simulink model "FDIBenchMark"  (Simulink 8.4)
settings: Solver=ode45  StartTime=0.0  StopTime=4400  FixedStep=Ts  RelTol=1e-12
InitFcn:
  | FDIBenchMarkData
values from neighbouring files (symbols this model uses):
  a = 2.2    [FDIBenchMarkData.m]
  Addt = [-(B_dt+B_r)/J_r B_dt/N_g/J_r -K_dt/J_r; eta_dt*B_dt/N_g/J_g -(eta_dt*B_dt/N_g^2+B_g)/J_g eta_dt*K_dt/N_g/J_g; 1 -1/N_g 0]    [FDIBenchMarkData.m]
  Addt2 = [-(B_dt+B_r)/J_r B_dt/N_g/J_r -K_dt/J_r; eta_dt2*B_dt/N_g/J_g -(eta_dt2*B_dt/N_g^2+B_g)/J_g eta_dt2*K_dt/N_g/J_g; 1 -1/N_g 0]    [FDIBenchMarkData.m]
  alpha = 0.1    [FDIBenchMarkData.m]
  alpha_gc = 50    [FDIBenchMarkData.m]
  Bddt = [1/J_r 0; 0 -1/J_g;0 0]    [FDIBenchMarkData.m]
  Bddt2 = [1/J_r 0; 0 -1/J_g;0 0]    [FDIBenchMarkData.m]
  Cddt = [1 0 0;0 1 0]    [FDIBenchMarkData.m]
  Constant_Beta_1_m1 = 5    [FDIBenchMarkData.m]
  Constant_Beta_3_m1 = 10    [FDIBenchMarkData.m]
  Constant_Omega_r_m1 = 1.4    [FDIBenchMarkData.m]
  Constant_tau_gc = 100    [FDIBenchMarkData.m]
  eta_gc = 0.98    [FDIBenchMarkData.m]
  Gain_Beta_2_m2 = 1.2    [FDIBenchMarkData.m]
  Gain_Omega_r_m2 = 1.1    [FDIBenchMarkData.m]
  H = 87    [FDIBenchMarkData.m]
  k = 4.7    [FDIBenchMarkData.m]
  K_i = 1    [FDIBenchMarkData.m]
  K_opt = .5* rho* pi*R^2*eta_dt*R^3*0.4554/(N_g*8)^3    (= 1.21708013189)    [FDIBenchMarkData.m]
  K_p = 4    [FDIBenchMarkData.m]
  L = acker(A', C', vpe)'    [FDIBenchMarkData.m]
  Lungime_Fereastra = 512    [FDIBenchMarkData.m]
  Lungime_Fereastra_2 = 5    [FDIBenchMarkData.m]
  Lungime_Fereastra_3 = 100    [FDIBenchMarkData.m]
  m = 1+alpha*(alpha-1)*R^2/(8*H^2)    (= 0.995085835315)    [FDIBenchMarkData.m]
  m_Beta = 0    [FDIBenchMarkData.m]
  m_omega_g = 0    [FDIBenchMarkData.m]
  m_omega_r = 0    [FDIBenchMarkData.m]
  m_P_g = 0    [FDIBenchMarkData.m]
  m_tau_g = 0    [FDIBenchMarkData.m]
  m_vw = 1.5    [FDIBenchMarkData.m]
  Omega_delta = 15    [FDIBenchMarkData.m]
  omega_n = 11.11    [FDIBenchMarkData.m]
  Omega_nom = 162    [FDIBenchMarkData.m]
  P_r = 4.8e6    (= 4800000)    [FDIBenchMarkData.m]
  R = 57.5    [FDIBenchMarkData.m]
  r = D_rotor/2    (= 57.5)    [FDIBenchMarkData.m]
  r0 = 1.5    [FDIBenchMarkData.m]
  rho = 1.225    [FDIBenchMarkData.m]
  seed = ceil(seed)    [FDIBenchMarkData.m]
  sigma_Beta = 0.2    [FDIBenchMarkData.m]
  sigma_omega_g = 0.05    [FDIBenchMarkData.m]
  sigma_omega_r = 0.004*2*pi    (= 0.0251327412287)    [FDIBenchMarkData.m]
  sigma_P_g = 1e3    (= 1000)    [FDIBenchMarkData.m]
  sigma_tau_g = 90    [FDIBenchMarkData.m]
  sigma_vm = 0.5    [FDIBenchMarkData.m]
  T_sample = 0.05    [FDIBenchMarkData.m]
  Ts = 1/100    (= 0.01)    [FDIBenchMarkData.m]
  turb_int = Turbulence_intensity    (= 12)    [FDIBenchMarkData.m]
  xi = 0.6    [FDIBenchMarkData.m]
undefined symbols (not defined in the file or in its folder): A, Apb, Apb1, Apb2, B, Bpb, Bpb1, Bpb2, C, Cpb, Cpb1, Cpb2, Cq, Fa, Fb, u0
undefined symbols (not defined in the file): turbulence_seeds
(part 1 of 2)
settings Model: Creator=peodg  LastModifiedBy=ALEXANDRU
settings SolverCC: MaxConsecutiveZCs=1e6
settings OptimizationCC: InitFltsAndDblsToZero=on
settings SFSimCC: SimParseCustomCode=off

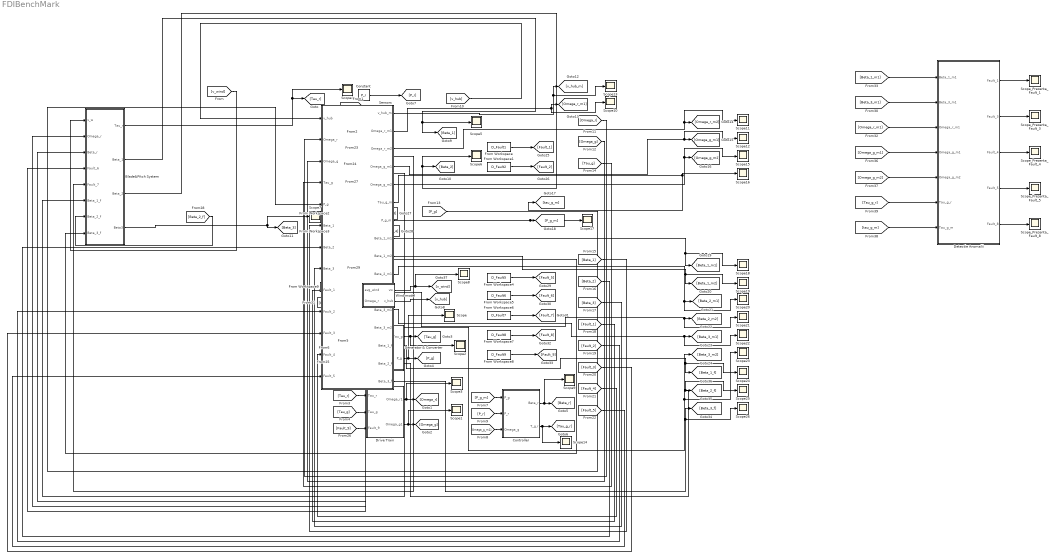
== system FDIBenchMark ==
  Blade&Pitch System : Subsystem
  Constant : Constant  Value=P_r
  Controller : Subsystem
  Detectie Anomalii : Subsystem
  Drive Train : Subsystem
  From Workspace : FromWorkspace  VariableName=D_Fault1  SampleTime=Ts
  From Workspace1 : FromWorkspace  VariableName=D_Fault2  SampleTime=Ts
  From Workspace2 : FromWorkspace  VariableName=D_Fault3  SampleTime=Ts
  From Workspace3 : FromWorkspace  VariableName=D_Fault4  SampleTime=Ts
  From Workspace4 : FromWorkspace  VariableName=D_Fault5  SampleTime=Ts
  From Workspace5 : FromWorkspace  VariableName=D_Fault6  SampleTime=Ts
  From Workspace6 : FromWorkspace  VariableName=D_Fault7  SampleTime=Ts
  From Workspace7 : FromWorkspace  VariableName=D_Fault8  SampleTime=Ts
  From Workspace8 : FromWorkspace  VariableName=D_Fault9  SampleTime=Ts
  From Workspace9 : FromWorkspace  VariableName=D_v_wind
  Generator & Converter : Subsystem
  Scope{,1..26} (27 alike) : Scope
      Scope settings: YMin=200000  YMax=1.2e+06  SaveName=P_g  SampleInput=on  SampleTime=Ts
      Scope1 settings: YMin=64  YMax=66.25  SaveName=Oemga_g1  SampleInput=on  SampleTime=Ts
      Scope10 settings: YMin=1.1  YMax=2.4  SaveName=Omega_r_m1  SampleInput=on  SampleTime=Ts
      Scope11 settings: YMin=-1  YMax=1  SaveName=Omega_r_m2  SampleInput=on  SampleTime=Ts
      Scope12 settings: YMin=-1  YMax=1  SaveName=Omega_g_m1  SampleInput=on  SampleTime=Ts
      Scope13 settings: YMin=-1  YMax=1  SaveName=v_hub_m  SampleInput=on  SampleTime=Ts
      Scope14 settings: YMin=-2.5  YMax=20  SaveName=T_g_r  SampleInput=on  SampleTime=Ts
      Scope15 settings: YMin=-1  YMax=1  SaveName=Omega_g_m2  SampleInput=on  SampleTime=Ts
      Scope16 settings: YMin=-1  YMax=1  SaveName=Tau_g_m  SampleInput=on  SampleTime=Ts
      Scope17 settings: YMin=-1  YMax=1  SaveName=P_g_m  SampleInput=on  SampleTime=Ts
      Scope18 settings: YMin=-1  YMax=1  SaveName=Beta_1_m1  SampleInput=on  SampleTime=Ts
      Scope19 settings: YMin=-1  YMax=1  SaveName=Beta_1_m2  SampleInput=on  SampleTime=Ts
      Scope2 settings: YMin=29400  YMax=29875  SaveName=Tau_g  SampleInput=on  SampleTime=Ts
      Scope20 settings: YMin=-1  YMax=1  SaveName=Beta_2_m1  SampleInput=on  SampleTime=Ts
      Scope21 settings: YMin=-1  YMax=1  SaveName=Beta_2_m2  SampleInput=on  SampleTime=Ts
      Scope22 settings: YMin=-1  YMax=1  SaveName=Beta_3_m1  SampleInput=on  SampleTime=Ts
      Scope23 settings: YMin=-1  YMax=1  SaveName=Beta_3_m2  SampleInput=on  SampleTime=Ts
      Scope24 settings: YMin=-1  YMax=1  SaveName=Beta_1_f  SampleInput=on  SampleTime=Ts
      Scope25 settings: YMin=-1  YMax=1  SaveName=Beta_2_f  SampleInput=on  SampleTime=Ts
      Scope26 settings: YMin=-1  YMax=1  SaveName=Beta_3_f  SampleInput=on  SampleTime=Ts
      Scope3 settings: YMin=0.62  YMax=0.69  SaveName=Omega_r1  SampleInput=on  SampleTime=Ts
      Scope4 settings: YMin=-1e+006  YMax=6e+006  SaveName=Tau_r  SampleInput=on  SampleTime=Ts
      Scope5 settings: YMin=-3  YMax=8  SaveName=Beta1  SampleInput=on  SampleTime=Ts
      Scope6 settings: YMin=-0.3  YMax=0.3  SaveName=Beta  SampleInput=on  SampleTime=Ts
      Scope7 settings: YMin=-0.25  YMax=0.35  SaveName=Beta3  SampleInput=on  SampleTime=Ts
      Scope8 settings: YMin=3  YMax=18  SaveName=Vw  SampleInput=on  SampleTime=Ts
      Scope9 settings: YMin=-1  YMax=1  SaveName=Beta_r  SampleInput=on  SampleTime=Ts
  Scope_Prezenta_Fault_{1,3..5,8} (5 alike) : Scope
      Scope_Prezenta_Fault_1 settings: YMin=-0  YMax=2  SaveName=ScopeData5
      Scope_Prezenta_Fault_3 settings: YMin=-0.03  YMax=0.02
      Scope_Prezenta_Fault_4 settings: YMin=-0.03  YMax=0.02
      Scope_Prezenta_Fault_5 settings: YMin=-0.03  YMax=0.02  SaveName=ScopeData8
      Scope_Prezenta_Fault_8 settings: YMin=-0.03  YMax=0.02  SaveName=ScopeData9
  Sensors : Subsystem
  Wind model : Subsystem
  wires:
  [v_wind] -> Blade&Pitch System/1(v_w)
  [Omega_r] -> Blade&Pitch System/2(Omega_r)
  [Beta_r] -> Blade&Pitch System/3(Beta_r)
  [Tau_r] -> Drive Train/1(Tau_r)
  [Tau_g] -> Drive Train/2(Tau_g)
  Drive Train/1(Omega_r1) -> [Omega_r], Scope3/1
  [Tau_g_r] -> Generator & Converter/1(Tau_g,r)
  [Omega_g] -> Generator & Converter/2(Omega_g)
  Generator & Converter/1(Tau_g) -> [Tau_g], Scope2/1
  Generator & Converter/2(P_g) -> [P_g], Scope/1
  [P_g_m] -> Controller/1(P_g)
  [Omega_g_m1] -> Controller/3(Omega_g)
  Controller/1(Beta_r) -> [Beta_r], Scope9/1
  Controller/2(T_g,r) -> [Tau_g_r], Scope14/1
  [P_r] -> Controller/2(P_r)
  Constant/1 -> [P_r]
  Sensors/1(v_hub_m) -> [v_hub_m], Scope13/1
  Sensors/2(Omega_r_m1) -> [Omega_r_m1], Scope10/1
  Sensors/3(Omega_r_m2) -> [Omega_r_m2], Scope11/1
  Sensors/4(Omega_g_m1) -> [Omega_g_m1], Scope12/1
  Sensors/5(Omega_g_m2) -> Scope15/1, [Omega_g_m2]
  Sensors/6(Tau_g_m) -> [tau_g_m], Scope16/1
  Sensors/7(P_g_m) -> [P_g_m], Scope17/1
  Sensors/8(Beta_1_m1) -> [Beta_1_m1], Scope18/1
  Sensors/9(Beta_1_m2) -> [Beta_1_m2], Scope19/1
  Sensors/10(Beta_2_m1) -> [Beta_2_m1], Scope20/1
  Sensors/11(Beta_2_m2) -> [Beta_2_m2], Scope21/1
  Sensors/12(Beta_3_m1) -> [Beta_3_m1], Scope22/1
  Sensors/13(Beta_3_m2) -> [Beta_3_m2], Scope23/1
  [v_hub] -> Sensors/1(v_hub)
  [Omega_r] -> Sensors/2(Omega_r)
  [Omega_g] -> Sensors/3(Omega_g)
  [Tau_g] -> Sensors/4(Tau_g)
  [P_g] -> Sensors/5(P_g)
  [Beta_1] -> Sensors/6(Beta_1)
  [Beta_2] -> Sensors/7(Beta_2)
  [Beta_3] -> Sensors/8(Beta_3)
  [Fault_1] -> Sensors/9(Fault_1)
  [Fault_2] -> Sensors/10(Fault_2)
  [Fault_3] -> Sensors/11(Fault_3)
  [Fault_4] -> Sensors/12(Fault_4)
  [Fault_5] -> Sensors/13(Fault_5)
  [Fault_6] -> Blade&Pitch System/4(Fault_6)
  [Fault_7] -> Blade&Pitch System/5(Fault_7)
  [Fault_8] -> Generator & Converter/3(Fault_8)
  [Fault_9] -> Drive Train/3(Fault_9)
  From Workspace8/1 -> [Fault_9]
  From Workspace7/1 -> [Fault_8]
  From Workspace6/1 -> [Fault_7]
  From Workspace5/1 -> [Fault_6]
  From Workspace4/1 -> [Fault_5]
  From Workspace3/1 -> [Fault_4]
  From Workspace2/1 -> [Fault_3]
  From Workspace1/1 -> [Fault_2]
  From Workspace/1 -> [Fault_1]
  Drive Train/2(Omega_g1) -> [Omega_g], Scope1/1
  Sensors/16(Beta_3_f) -> [Beta_3_f], Scope26/1
  Sensors/15(Beta_2_f) -> [Beta_2_f], Scope25/1
  Sensors/14(Beta_1_f) -> [Beta_1_f], Scope24/1
  [Beta_1_f] -> Blade&Pitch System/6(Beta_1_f)
  [Beta_2_f] -> Blade&Pitch System/7(Beta_2_f)
  [Beta_3_f] -> Blade&Pitch System/8(Beta_3_f)
  Blade&Pitch System/4(Beta3) -> [Beta_3], Scope7/1
  Blade&Pitch System/3(Beta_2) -> [Beta_2], Scope6/1
  Blade&Pitch System/2(Beta_1) -> [Beta_1], Scope5/1
  Blade&Pitch System/1(Tau_r) -> [Tau_r], Scope4/1
  Wind model/1(vw) -> [v_wind], Scope8/1
  Wind model/2(v_hub) -> [v_hub]
  [Omega_r] -> Wind model/2(Omega_r)
  From Workspace9/1 -> Wind model/1(avg_wind)
  [Beta_1_m1] -> Detectie Anomalii/1(Beta_1_m1)
  [Beta_3_m1] -> Detectie Anomalii/2(Beta_3_m1)
  [Omega_r_m1] -> Detectie Anomalii/3(Omega_r_m1)
  [Omega_g_m1] -> Detectie Anomalii/4(Omega_g_m1)
  [Omega_g_m2] -> Detectie Anomalii/5(Omega_g_m2)
  [Tau_g_r] -> Detectie Anomalii/6(Tau_g_r)
  [tau_g_m] -> Detectie Anomalii/7(Tau_g_m)
  Detectie Anomalii/1(Fault_1) -> Scope_Prezenta_Fault_1/1
  Detectie Anomalii/2(Fault_3) -> Scope_Prezenta_Fault_3/1
  Detectie Anomalii/3(Fault_4) -> Scope_Prezenta_Fault_4/1
  Detectie Anomalii/4(Fault_5) -> Scope_Prezenta_Fault_5/1
  Detectie Anomalii/5(Fault_8) -> Scope_Prezenta_Fault_8/1

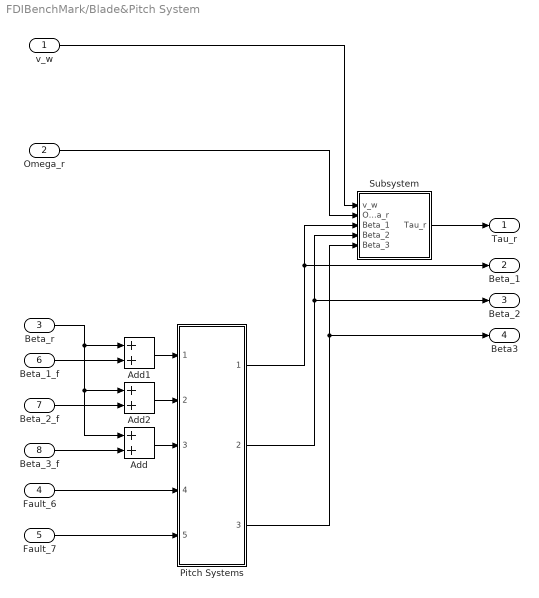
== system FDIBenchMark/Blade&Pitch System ==
  v_w : Inport
  Omega_r : Inport  Port=2
  Beta_r : Inport  Port=3
  Fault_6 : Inport  Port=4
  Fault_7 : Inport  Port=5
  Beta_1_f : Inport  Port=6
  Beta_2_f : Inport  Port=7
  Beta_3_f : Inport  Port=8
  Add : Sum
  Add1 : Sum
  Add2 : Sum
  Pitch Systems : Subsystem
  Subsystem : Subsystem
  Tau_r : Outport
  Beta_1 : Outport  Port=2
  Beta_2 : Outport  Port=3
  Beta3 : Outport  Port=4
  wires:
  Pitch Systems/1(Beta_1) -> Subsystem/3(Beta_1), Beta_1/1
  Pitch Systems/2(Beta_2) -> Subsystem/4(Beta_2), Beta_2/1
  Pitch Systems/3(Beta_3) -> Subsystem/5(Beta_3), Beta3/1
  Subsystem/1(Tau_r) -> Tau_r/1
  v_w/1 -> Subsystem/1(v_w)
  Omega_r/1 -> Subsystem/2(Omega_r)
  Fault_6/1 -> Pitch Systems/4(Fault_6)
  Fault_7/1 -> Pitch Systems/5(Fault_7)
  Add/1 -> Pitch Systems/3(Beta_r3)
  Add1/1 -> Pitch Systems/1(Beta_r1)
  Add2/1 -> Pitch Systems/2(Beta_r2)
  Beta_3_f/1 -> Add/2
  Beta_2_f/1 -> Add2/2
  Beta_1_f/1 -> Add1/2
  Beta_r/1 -> Add1/1, Add2/1, Add/1

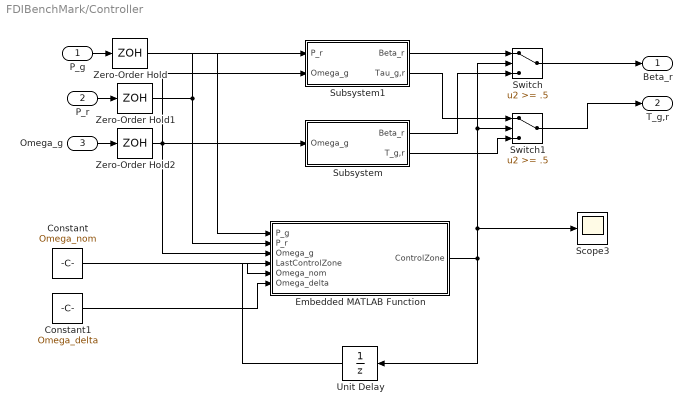
== system FDIBenchMark/Controller ==
  P_g : Inport
  P_r : Inport  Port=2
  Omega_g : Inport  Port=3
  Constant : Constant  Value=Omega_nom
  Constant1 : Constant  Value=Omega_delta
  Embedded MATLAB Function : MATLAB Function  TreatAsAtomicUnit=on
  Scope3 : Scope
      settings: YMin=0.62  YMax=0.69  SaveName=Omega_r  SampleInput=on  SampleTime=Ts
  Subsystem : Subsystem
  Subsystem1 : Subsystem
  Switch : Switch  Threshold=.5
  Switch1 : Switch  Threshold=.5
  Unit Delay : UnitDelay  SampleTime=Ts
  Zero-Order Hold : ZeroOrderHold  SampleTime=Ts
  Zero-Order Hold1 : ZeroOrderHold  SampleTime=Ts
  Zero-Order Hold2 : ZeroOrderHold  SampleTime=Ts
  Beta_r : Outport
  T_g,r : Outport  Port=2
  wires:
  Embedded MATLAB Function/1(ControlZone) -> Unit Delay/1, Switch/2, Switch1/2, Scope3/1
  Unit Delay/1 -> Embedded MATLAB Function/4(LastControlZone)
  P_g/1 -> Zero-Order Hold/1
  P_r/1 -> Zero-Order Hold1/1
  Omega_g/1 -> Zero-Order Hold2/1
  Switch/1 -> Beta_r/1
  Switch1/1 -> T_g,r/1
  Subsystem1/1(Beta_r) -> Switch/1
  Subsystem/1(Beta_r) -> Switch/3
  Subsystem1/2(Tau_g,r) -> Switch1/1
  Subsystem/2(T_g,r) -> Switch1/3
  Constant/1 -> Embedded MATLAB Function/5(Omega_nom)
  Constant1/1 -> Embedded MATLAB Function/6(Omega_delta)
  Zero-Order Hold/1 -> Embedded MATLAB Function/1(P_g)
  Zero-Order Hold1/1 -> Subsystem1/1(P_r), Embedded MATLAB Function/2(P_r)
  Zero-Order Hold2/1 -> Embedded MATLAB Function/3(Omega_g), Subsystem1/2(Omega_g), Subsystem/1(Omega_g)

== system FDIBenchMark/Detectie Anomalii ==
  Beta_1_m1 : Inport
  Beta_3_m1 : Inport  Port=2
  Omega_r_m1 : Inport  Port=3
  Omega_g_m1 : Inport  Port=4
  Omega_g_m2 : Inport  Port=5
  Tau_g_r : Inport  Port=6
  Tau_g_m : Inport  Port=7
  Detectie Fault_1 : Subsystem
  Detectie Fault_3 : Subsystem
  Detectie Fault_4 : Subsystem
  Detectie Fault_5 : Subsystem
  Detectie Fault_8 : Subsystem
  Fault_1 : Outport
  Fault_3 : Outport  Port=2
  Fault_4 : Outport  Port=3
  Fault_5 : Outport  Port=4
  Fault_8 : Outport  Port=5
  wires:
  Tau_g_m/1 -> Detectie Fault_8/2(Tau_g_m)
  Omega_g_m2/1 -> Detectie Fault_5/2(Omega_g_m2)
  Detectie Fault_5/1(Prezenta_Fault_5) -> Fault_5/1
  Omega_g_m1/1 -> Detectie Fault_5/1(Omega_g_m1)
  Beta_1_m1/1 -> Detectie Fault_1/1(Beta_1_m1)
  Detectie Fault_3/1(Prezenta_Fault_3) -> Fault_3/1
  Detectie Fault_4/1(Prezenta_Fault_4) -> Fault_4/1
  Omega_r_m1/1 -> Detectie Fault_4/1(Omega_r_m1)
  Detectie Fault_1/1(Prezenta_Fault_1) -> Fault_1/1
  Beta_3_m1/1 -> Detectie Fault_3/1(Beta_3_m1)
  Detectie Fault_8/1(Prezenta_Fault_8) -> Fault_8/1
  Tau_g_r/1 -> Detectie Fault_8/1(Tau_g_r)

== system FDIBenchMark/Drive Train ==
  Tau_r : Inport
  Tau_g : Inport  Port=2
  Fault_9 : Inport  Port=3
  Add : Sum
  Demux1 : Demux  Outputs=2
  Gain : Gain  Gain=Addt  Multiplication=Matrix(K*u)
  Gain1 : Gain  Gain=Bddt  Multiplication=Matrix(K*u)
  Gain2 : Gain  Gain=Cddt  Multiplication=Matrix(K*u)
  Gain3 : Gain  Gain=Addt2  Multiplication=Matrix(K*u)
  Gain4 : Gain  Gain=Bddt2  Multiplication=Matrix(K*u)
  Integrator : Integrator  InitialCondition=[1 100 0]
  Mux : Mux  Inputs=2
  Switch1 : Switch  Threshold=0.5
  Switch2 : Switch  Threshold=0.5
  Omega_r1 : Outport
  Omega_g1 : Outport  Port=2
  wires:
  Tau_r/1 -> Mux/1
  Tau_g/1 -> Mux/2
  Integrator/1 -> Gain2/1, Gain/1, Gain3/1
  Add/1 -> Integrator/1
  Switch1/1 -> Add/1
  Gain1/1 -> Switch1/1
  Gain4/1 -> Switch1/3
  Gain/1 -> Switch2/1
  Gain3/1 -> Switch2/3
  Switch2/1 -> Add/2
  Demux1/1 -> Omega_r1/1
  Demux1/2 -> Omega_g1/1
  Gain2/1 -> Demux1/1
  Fault_9/1 -> Switch1/2, Switch2/2
  Mux/1 -> Gain1/1, Gain4/1

== system FDIBenchMark/Generator & Converter ==
  Tau_g,r : Inport
  Omega_g : Inport  Port=2
  Fault_8 : Inport  Port=3
  Bias : Bias  Bias=Constant_tau_gc
  Divide : Product  Inputs=**
  Gain : Gain  Gain=eta_gc
  Switch : Switch  Threshold=0.5
  Transfer Fcn : TransferFcn  Numerator=[alpha_gc]  Denominator=[1 alpha_gc]
  Tau_g : Outport
  P_g : Outport  Port=2
  wires:
  Tau_g,r/1 -> Transfer Fcn/1
  Gain/1 -> P_g/1
  Divide/1 -> Gain/1
  Omega_g/1 -> Divide/2
  Transfer Fcn/1 -> Bias/1, Switch/1
  Fault_8/1 -> Switch/2
  Switch/1 -> Divide/1, Tau_g/1
  Bias/1 -> Switch/3

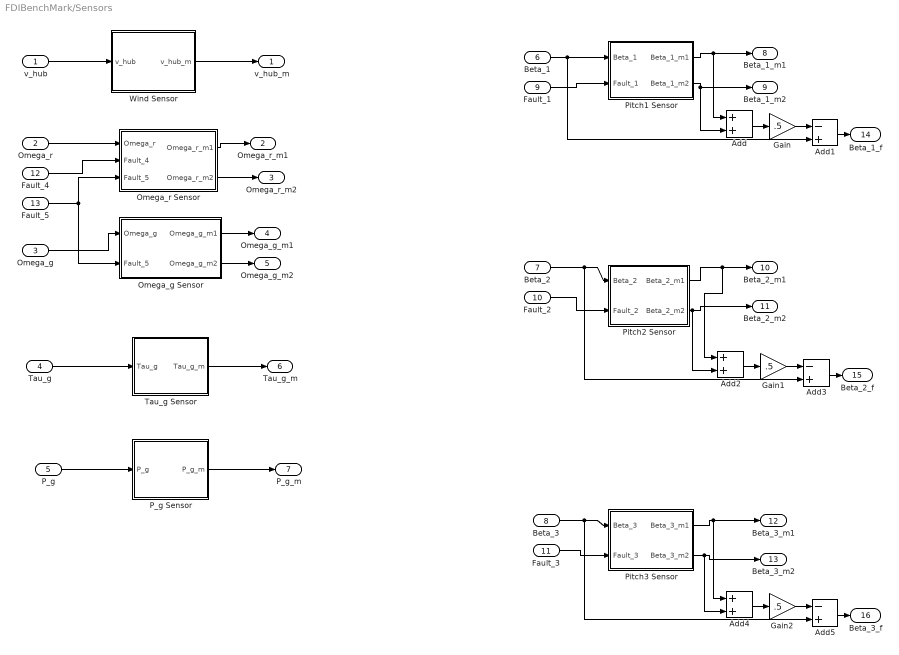
== system FDIBenchMark/Sensors ==
  v_hub : Inport
  Omega_r : Inport  Port=2
  Omega_g : Inport  Port=3
  Tau_g : Inport  Port=4
  P_g : Inport  Port=5
  Beta_1 : Inport  Port=6
  Beta_2 : Inport  Port=7
  Beta_3 : Inport  Port=8
  Fault_1 : Inport  Port=9
  Fault_2 : Inport  Port=10
  Fault_3 : Inport  Port=11
  Fault_4 : Inport  Port=12
  Fault_5 : Inport  Port=13
  Add : Sum
  Add1 : Sum  Inputs=-+
  Add2 : Sum
  Add3 : Sum  Inputs=-+
  Add4 : Sum
  Add5 : Sum  Inputs=-+
  Gain : Gain  Gain=.5
  Gain1 : Gain  Gain=.5
  Gain2 : Gain  Gain=.5
  Omega_g Sensor : Subsystem
  Omega_r Sensor : Subsystem
  P_g Sensor : Subsystem
  Pitch1 Sensor : Subsystem
  Pitch2 Sensor : Subsystem
  Pitch3 Sensor : Subsystem
  Tau_g Sensor : Subsystem
  Wind Sensor : Subsystem
  v_hub_m : Outport
  Omega_r_m1 : Outport  Port=2
  Omega_r_m2 : Outport  Port=3
  Omega_g_m1 : Outport  Port=4
  Omega_g_m2 : Outport  Port=5
  Tau_g_m : Outport  Port=6
  P_g_m : Outport  Port=7
  Beta_1_m1 : Outport  Port=8
  Beta_1_m2 : Outport  Port=9
  Beta_2_m1 : Outport  Port=10
  Beta_2_m2 : Outport  Port=11
  Beta_3_m1 : Outport  Port=12
  Beta_3_m2 : Outport  Port=13
  Beta_1_f : Outport  Port=14
  Beta_2_f : Outport  Port=15
  Beta_3_f : Outport  Port=16
  wires:
  Wind Sensor/1(v_hub_m) -> v_hub_m/1
  v_hub/1 -> Wind Sensor/1(v_hub)
  Omega_r/1 -> Omega_r Sensor/1(Omega_r)
  Omega_r Sensor/1(Omega_r_m1) -> Omega_r_m1/1
  Omega_r Sensor/2(Omega_r_m2) -> Omega_r_m2/1
  Omega_g/1 -> Omega_g Sensor/1(Omega_g)
  Omega_g Sensor/1(Omega_g_m1) -> Omega_g_m1/1
  Omega_g Sensor/2(Omega_g_m2) -> Omega_g_m2/1
  Tau_g/1 -> Tau_g Sensor/1(Tau_g)
  Tau_g Sensor/1(Tau_g_m) -> Tau_g_m/1
  P_g/1 -> P_g Sensor/1(P_g)
  P_g Sensor/1(P_g_m) -> P_g_m/1
  Beta_1/1 -> Pitch1 Sensor/1(Beta_1), Add1/2
  Pitch1 Sensor/1(Beta_1_m1) -> Beta_1_m1/1, Add/1
  Pitch1 Sensor/2(Beta_1_m2) -> Beta_1_m2/1, Add/2
  Beta_2/1 -> Pitch2 Sensor/1(Beta_2), Add3/2
  Pitch2 Sensor/1(Beta_2_m1) -> Beta_2_m1/1, Add2/1
  Pitch2 Sensor/2(Beta_2_m2) -> Beta_2_m2/1, Add2/2
  Beta_3/1 -> Pitch3 Sensor/1(Beta_3), Add5/2
  Pitch3 Sensor/1(Beta_3_m1) -> Beta_3_m1/1, Add4/1
  Pitch3 Sensor/2(Beta_3_m2) -> Beta_3_m2/1, Add4/2
  Fault_1/1 -> Pitch1 Sensor/2(Fault_1)
  Fault_2/1 -> Pitch2 Sensor/2(Fault_2)
  Fault_3/1 -> Pitch3 Sensor/2(Fault_3)
  Fault_4/1 -> Omega_r Sensor/2(Fault_4)
  Fault_5/1 -> Omega_r Sensor/3(Fault_5), Omega_g Sensor/2(Fault_5)
  Add/1 -> Gain/1
  Gain/1 -> Add1/1
  Add1/1 -> Beta_1_f/1
  Add2/1 -> Gain1/1
  Gain1/1 -> Add3/1
  Add3/1 -> Beta_2_f/1
  Add4/1 -> Gain2/1
  Gain2/1 -> Add5/1
  Add5/1 -> Beta_3_f/1

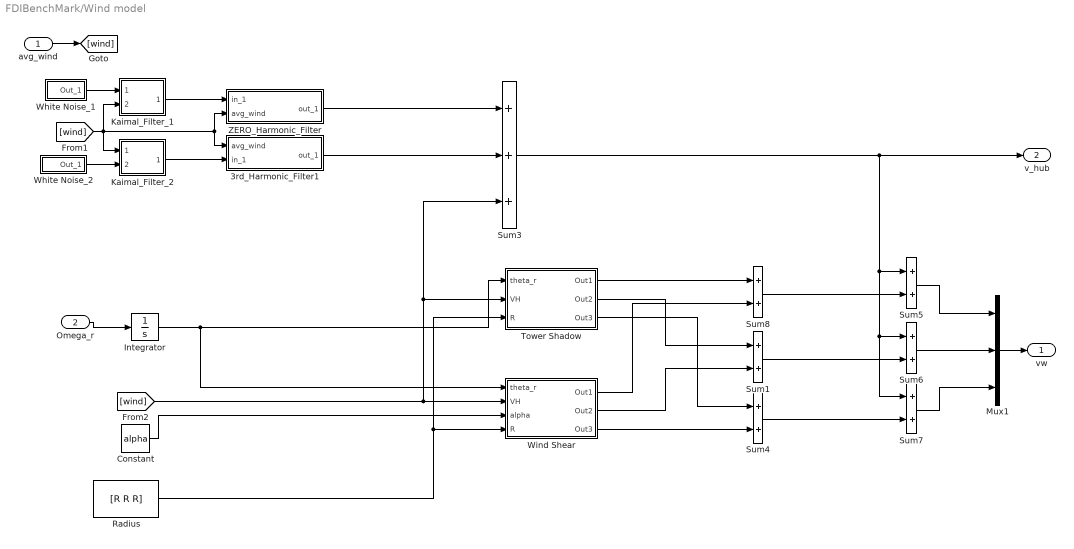
== system FDIBenchMark/Wind model ==
  avg_wind : Inport
  Omega_r : Inport  Port=2
  3rd_Harmonic_Filter1 : Subsystem
  Constant : Constant  Value=alpha
  Integrator : Integrator
  Kaimal_Filter_1 : Subsystem
  Kaimal_Filter_2 : Subsystem
  Mux1 : Mux  Inputs=3
  Radius : Constant  Value=[R R R]
  Sum{1,4..8} (6 alike) : Sum  SaturateOnIntegerOverflow=on  InputSameDT=on  OutDataTypeStr=Inherit: Same as first input
  Sum3 : Sum  Inputs=+++  SaturateOnIntegerOverflow=on  InputSameDT=on  OutDataTypeStr=Inherit: Same as first input
  Tower Shadow : Subsystem
  White Noise_1 : Subsystem  mask(Continuous White Noise.){Cov=[1], Ts=T_sample, seed=turbulence_seeds(1)}
      mask prompts: Cov "Noise Power:"; Ts "Sample Time:"
      mask help:
      | White noise for continuous (s-domain) systems.
      | Band-limited using zero-order-hold.
      mask init:
      | r = rand(1,12); r2 = [r(1),r;r,r(12)]; t =[1:13;1:13];
      mask Help: Implemented using white noise into Zero-Order Hold block. The seed and power can be vectors of the same length to produce a vector of white noise sources. For faster simulation, set sample time to the highest value possible but in accordance with the fastest dynamics of system.
      mask Display: plot(t(:),r2(:))
  White Noise_2 : Subsystem  mask(Continuous White Noise.){Cov=[1], Ts=T_sample, seed=turbulence_seeds(2)}
      mask prompts: Cov "Noise Power:"; Ts "Sample Time:"
      mask help:
      | White noise for continuous (s-domain) systems.
      | Band-limited using zero-order-hold.
      mask init:
      | r = rand(1,12); r2 = [r(1),r;r,r(12)]; t =[1:13;1:13];
      mask Help: Implemented using white noise into Zero-Order Hold block. The seed and power can be vectors of the same length to produce a vector of white noise sources. For faster simulation, set sample time to the highest value possible but in accordance with the fastest dynamics of system.
      mask Display: plot(t(:),r2(:))
  Wind Shear : Subsystem
  ZERO_Harmonic_Filter : Subsystem
  vw : Outport  InitialOutput=[u0]
  v_hub : Outport  Port=2  InitialOutput=[u0]
  wires:
  [wind] -> 3rd_Harmonic_Filter1/1(avg_wind), ZERO_Harmonic_Filter/2(avg_wind), Kaimal_Filter_2/1(avg_wind), Kaimal_Filter_1/2(avg_wind)
  avg_wind/1 -> [wind]
  White Noise_2/1(Out_1) -> Kaimal_Filter_2/2(in_1)
  Kaimal_Filter_2/1(out_1) -> 3rd_Harmonic_Filter1/2(in_1)
  Kaimal_Filter_1/1(out_1) -> ZERO_Harmonic_Filter/1(in_1)
  White Noise_1/1(Out_1) -> Kaimal_Filter_1/1(in_1)
  [wind] -> Wind Shear/2(VH), Sum3/3, Tower Shadow/2(VH)
  Constant/1 -> Wind Shear/3(alpha)
  Radius/1 -> Wind Shear/4(R), Tower Shadow/3(R)
  Tower Shadow/1(Out1) -> Sum8/1
  Wind Shear/1(Out1) -> Sum8/2
  Tower Shadow/2(Out2) -> Sum1/1
  Wind Shear/2(Out2) -> Sum1/2
  Tower Shadow/3(Out3) -> Sum4/1
  Wind Shear/3(Out3) -> Sum4/2
  Sum8/1 -> Sum5/2
  Sum1/1 -> Sum6/2
  Sum4/1 -> Sum7/2
  Sum5/1 -> Mux1/1
  Sum6/1 -> Mux1/2
  Sum7/1 -> Mux1/3
  Mux1/1 -> vw/1
  Sum3/1 -> Sum6/1, Sum7/1, Sum5/1, v_hub/1
  3rd_Harmonic_Filter1/1(out_1) -> Sum3/2
  ZERO_Harmonic_Filter/1(out_1) -> Sum3/1
  Omega_r/1 -> Integrator/1
  Integrator/1 -> Tower Shadow/1(theta_r), Wind Shear/1(theta_r)

== system FDIBenchMark/Blade&Pitch System/Pitch Systems ==
  Beta_r1 : Inport
  Beta_r2 : Inport  Port=2
  Beta_r3 : Inport  Port=3
  Fault_6 : Inport  Port=4
  Fault_7 : Inport  Port=5
  PitchSystem 1 : Subsystem
  PitchSystem 2 : Subsystem
  PitchSystem 3 : Subsystem
  Beta_1 : Outport
  Beta_2 : Outport  Port=2
  Beta_3 : Outport  Port=3
  wires:
  PitchSystem 1/1(Beta_1) -> Beta_1/1
  PitchSystem 2/1(Beta_2) -> Beta_2/1
  PitchSystem 3/1(Beta_3) -> Beta_3/1
  Fault_7/1 -> PitchSystem 3/2(Fault_7)
  Fault_6/1 -> PitchSystem 2/2(Fault_6)
  Beta_r3/1 -> PitchSystem 3/1(Beta_r)
  Beta_r2/1 -> PitchSystem 2/1(Beta_r)
  Beta_r1/1 -> PitchSystem 1/1(Beta_r)

== system FDIBenchMark/Blade&Pitch System/Subsystem ==
  v_w : Inport
  Omega_r : Inport  Port=2
  Beta_1 : Inport  Port=3
  Beta_2 : Inport  Port=4
  Beta_3 : Inport  Port=5
  Add : Sum  Inputs=+++
  AeroDyn 1 : Subsystem
  AeroDyn 2 : Subsystem
  AeroDyn 3 : Subsystem
  Demux : Demux  Outputs=3
  Scope1 : Scope
      settings: YMin=0.5225  YMax=0.545  SaveName=ScopeData12
  Scope3 : Scope
      settings: YMin=5  YMax=7.75  SaveName=ScopeData11
  Tau_r : Outport
  wires:
  Omega_r/1 -> AeroDyn 1/2(Omega_r), AeroDyn 3/2(Omega_r), AeroDyn 2/2(Omega_r), Scope1/1
  AeroDyn 1/1(Tau_r1) -> Add/1
  AeroDyn 2/1(Tau_r2) -> Add/2
  AeroDyn 3/1(Tau_r3) -> Add/3
  Beta_1/1 -> AeroDyn 1/3(Beta_1)
  Add/1 -> Tau_r/1
  Beta_2/1 -> AeroDyn 2/3(Beta_2)
  Beta_3/1 -> AeroDyn 3/3(Beta_3)
  v_w/1 -> Demux/1, Scope3/1
  Demux/3 -> AeroDyn 3/1(v_w)
  Demux/2 -> AeroDyn 2/1(v_w)
  Demux/1 -> AeroDyn 1/1(v_w)

== system FDIBenchMark/Controller/Subsystem ==
  Omega_g : Inport
  Constant : Constant  Value=0
  Gain : Gain  Gain=K_opt
  Product : Product  RndMeth=Zero
  Beta_r : Outport
  T_g,r : Outport  Port=2
  wires:
  Constant/1 -> Beta_r/1
  Omega_g/1 -> Product/2, Product/1
  Gain/1 -> T_g,r/1
  Product/1 -> Gain/1

== system FDIBenchMark/Controller/Subsystem1 ==
  P_r : Inport
  Omega_g : Inport  Port=2
  Add : Sum
  Bias : Bias  Bias=-Omega_nom
  Discrete-Time Integrator : DiscreteIntegrator  SampleTime=Ts  LimitOutput=on  UpperSaturationLimit=90  LowerSaturationLimit=-2
  Divide : Product  Inputs=/*
  Gain : Gain  Gain=K_p
  Gain1 : Gain  Gain=K_i
  Gain2 : Gain  Gain=1/eta_gc
  Saturation : Saturate  UpperLimit=90  LowerLimit=-2
  Beta_r : Outport
  Tau_g,r : Outport  Port=2
  wires:
  Divide/1 -> Gain2/1
  P_r/1 -> Divide/2
  Omega_g/1 -> Divide/1, Bias/1
  Bias/1 -> Discrete-Time Integrator/1, Gain/1
  Discrete-Time Integrator/1 -> Gain1/1
  Gain1/1 -> Add/2
  Gain/1 -> Add/1
  Add/1 -> Saturation/1
  Saturation/1 -> Beta_r/1
  Gain2/1 -> Tau_g,r/1

== system FDIBenchMark/Detectie Anomalii/Detectie Fault_1 ==
  Beta_1_m1 : Inport
  Calcul FFT : Subsystem
  Calcul Medie : Subsystem
  Decizie Fault_1 : Subsystem
  Ferestruire Semnal : Subsystem
  Ferestruire si Suprapunere Semnal : Subsystem
  Prezenta_Fault_1 : Outport
  wires:
  Beta_1_m1/1 -> Ferestruire si Suprapunere Semnal/1(Intrare_Semnal), Ferestruire Semnal/1(Intrare_Semnal)
  Calcul Medie/1(Iesire_Valoare) -> Decizie Fault_1/1(Intrare_Valoare_Medie)
  Ferestruire si Suprapunere Semnal/1(Iesire_Semnal) -> Calcul FFT/1(Intrare_Semnal)
  Calcul FFT/1(Iesire_Matrice) -> Decizie Fault_1/2(Intrare_Matrice_FFT)
  Decizie Fault_1/1(Iesire_Decizie) -> Prezenta_Fault_1/1
  Ferestruire Semnal/1(Iesire_Semnal) -> Calcul Medie/1(Intrare_Semnal)

== system FDIBenchMark/Detectie Anomalii/Detectie Fault_3 ==
  Beta_3_m1 : Inport
  Calcul FFT : Subsystem
  Calcul Medie : Subsystem
  Decizie Fault_3 : Subsystem
  Ferestruire Semnal : Subsystem
  Ferestruire si Suprapunere Semnal : Subsystem
  Prezenta_Fault_3 : Outport
  wires:
  Beta_3_m1/1 -> Ferestruire si Suprapunere Semnal/1(Intrare_Semnal), Ferestruire Semnal/1(Intrare_Semnal)
  Calcul Medie/1(Iesire_Valoare) -> Decizie Fault_3/1(Intrare_Valoare_Medie)
  Ferestruire si Suprapunere Semnal/1(Iesire_Semnal) -> Calcul FFT/1(Intrare_Semnal)
  Calcul FFT/1(Iesire_Matrice) -> Decizie Fault_3/2(Intrare_Matrice_FFT)
  Decizie Fault_3/1(Iesire_Decizie) -> Prezenta_Fault_3/1
  Ferestruire Semnal/1(Iesire_Semnal) -> Calcul Medie/1(Intrare_Semnal)

== system FDIBenchMark/Detectie Anomalii/Detectie Fault_4 ==
  Omega_r_m1 : Inport
  Calcul FFT : Subsystem
  Calcul Medie : Subsystem
  Decizie Fault_4 : Subsystem
  Ferestruire Semnal : Subsystem
  Ferestruire si Suprapunere Semnal : Subsystem
  Prezenta_Fault_4 : Outport
  wires:
  Omega_r_m1/1 -> Ferestruire si Suprapunere Semnal/1(Intrare_Semnal), Ferestruire Semnal/1(Intrare_Semnal)
  Calcul Medie/1(Iesire_Valoare) -> Decizie Fault_4/1(Intrare_Valoare_Medie)
  Ferestruire si Suprapunere Semnal/1(Iesire_Semnal) -> Calcul FFT/1(Intrare_Semnal)
  Calcul FFT/1(Iesire_Matrice) -> Decizie Fault_4/2(Intrare_Matrice_FFT)
  Decizie Fault_4/1(Iesire_Decizie) -> Prezenta_Fault_4/1
  Ferestruire Semnal/1(Iesire_Semnal) -> Calcul Medie/1(Intrare_Semnal)

== system FDIBenchMark/Detectie Anomalii/Detectie Fault_5 ==
  Omega_g_m1 : Inport
  Omega_g_m2 : Inport  Port=2
  Calcul Autocorelatie : Subsystem
  Calcul Autocorelatie1 : Subsystem
  Calcul Diferenta in Modul : Subsystem
  Calcul Maxim : Subsystem
  Decizie Fault_5 : Subsystem
  Ferestruire Semnal : Subsystem
  Ferestruire Semnal1 : Subsystem
  Prezenta_Fault_5 : Outport
  wires:
  Ferestruire Semnal/1(Iesire_Semnal) -> Calcul Autocorelatie/1(Intrare_Semnal)
  Calcul Autocorelatie/1(Iesire_Vector) -> Calcul Diferenta in Modul/1(Intrare_Vector_1)
  Calcul Autocorelatie1/1(Iesire_Vector) -> Calcul Diferenta in Modul/2(Intrare_Vector_2)
  Calcul Diferenta in Modul/1(Iesire_Vector) -> Calcul Maxim/1(Intrare_Vector)
  Calcul Maxim/1(Iesire_Valoare) -> Decizie Fault_5/1(Intrare_Valoare_Maxim)
  Decizie Fault_5/1(Iesire_Decizie) -> Prezenta_Fault_5/1
  Omega_g_m2/1 -> Ferestruire Semnal1/1(Intrare_Semnal)
  Omega_g_m1/1 -> Ferestruire Semnal/1(Intrare_Semnal)
  Ferestruire Semnal1/1(Iesire_Semnal) -> Calcul Autocorelatie1/1(Intrare_Semnal)

== system FDIBenchMark/Detectie Anomalii/Detectie Fault_8 ==
  Tau_g_r : Inport
  Tau_g_m : Inport  Port=2
  Calcul Reziduu : Subsystem
  Decizie Fault_8 : Subsystem
  Estimator : StateSpace  A=A-L*C  B=[B, L]  C=C  D=zeros(1,2)  X0=0
  Filtru : DiscreteFilter  Numerator=Fb  Denominator=Fa  SampleTime=Ts
  Matrix Concatenate2 : Concatenate  Mode=Multidimensional array
  Prezenta_Fault_8 : Outport
  wires:
  Filtru/1 -> Decizie Fault_8/1(Intrare_Reziduu_Filtrat)
  Matrix Concatenate2/1 -> Estimator/1
  Tau_g_m/1 -> Calcul Reziduu/1(Intrare_Semnal_Original), Matrix Concatenate2/2
  Decizie Fault_8/1(Iesire_Decizie) -> Prezenta_Fault_8/1
  Calcul Reziduu/1(Iesire_Reziduu) -> Filtru/1
  Tau_g_r/1 -> Matrix Concatenate2/1
  Estimator/1 -> Calcul Reziduu/2(Intrare_Semnal_Estimat)

== system FDIBenchMark/Sensors/Omega_g Sensor ==
  Omega_g : Inport
  Fault_5 : Inport  Port=2
  Add : Sum
  Add1 : Sum
  Gain : Gain  Gain=Gain_Omega_r_m2
  Random Number : RandomNumber  Mean=m_omega_g  Variance=sigma_omega_g  Seed=seed(4)  SampleTime=Ts
  Random Number1 : RandomNumber  Mean=m_omega_r  Variance=sigma_omega_r  Seed=seed(5)  SampleTime=Ts
  Switch1 : Switch  Threshold=0.5
  Omega_g_m1 : Outport
  Omega_g_m2 : Outport  Port=2
  wires:
  Random Number1/1 -> Add1/2
  Random Number/1 -> Add/1
  Omega_g/1 -> Add1/1, Add/2
  Add/1 -> Omega_g_m1/1
  Add1/1 -> Switch1/1, Gain/1
  Switch1/1 -> Omega_g_m2/1
  Fault_5/1 -> Switch1/2
  Gain/1 -> Switch1/3

== system FDIBenchMark/Sensors/Omega_r Sensor ==
  Omega_r : Inport
  Fault_4 : Inport  Port=2
  Fault_5 : Inport  Port=3
  Add : Sum
  Add1 : Sum
  Constant : Constant  Value=Constant_Omega_r_m1
  Gain : Gain  Gain=Gain_Omega_r_m2
  Random Number : RandomNumber  Mean=m_omega_r  Variance=sigma_omega_r  Seed=seed(2)  SampleTime=Ts
  Random Number1 : RandomNumber  Mean=m_omega_r  Variance=sigma_omega_r  Seed=seed(3)  SampleTime=Ts
  Switch : Switch  Threshold=0.5
  Switch1 : Switch  Threshold=0.5
  Omega_r_m1 : Outport
  Omega_r_m2 : Outport  Port=2
  wires:
  Omega_r/1 -> Add/2, Add1/1
  Random Number/1 -> Add/1
  Random Number1/1 -> Add1/2
  Fault_4/1 -> Switch/2
  Constant/1 -> Switch/3
  Add/1 -> Switch/1
  Switch/1 -> Omega_r_m1/1
  Add1/1 -> Switch1/1, Gain/1
  Switch1/1 -> Omega_r_m2/1
  Fault_5/1 -> Switch1/2
  Gain/1 -> Switch1/3

== system FDIBenchMark/Sensors/P_g Sensor ==
  P_g : Inport
  Add : Sum
  Random Number : RandomNumber  Mean=m_P_g  Variance=sigma_P_g  Seed=seed(7)  SampleTime=Ts
  P_g_m : Outport
  wires:
  Random Number/1 -> Add/2
  P_g/1 -> Add/1
  Add/1 -> P_g_m/1

== system FDIBenchMark/Sensors/Pitch1 Sensor ==
  Beta_1 : Inport
  Fault_1 : Inport  Port=2
  Add : Sum
  Add1 : Sum
  Constant : Constant  Value=Constant_Beta_1_m1
  Random Number : RandomNumber  Mean=m_Beta  Variance=sigma_Beta  Seed=seed(8)  SampleTime=Ts
  Random Number1 : RandomNumber  Mean=m_Beta  Variance=sigma_Beta  Seed=seed(9)  SampleTime=Ts
  Switch : Switch  Threshold=0.5
  Beta_1_m1 : Outport
  Beta_1_m2 : Outport  Port=2
  wires:
  Random Number1/1 -> Add1/2
  Add1/1 -> Beta_1_m2/1
  Random Number/1 -> Add/1
  Beta_1/1 -> Add1/1, Add/2
  Fault_1/1 -> Switch/2
  Constant/1 -> Switch/3
  Add/1 -> Switch/1
  Switch/1 -> Beta_1_m1/1

== system FDIBenchMark/Sensors/Pitch2 Sensor ==
  Beta_2 : Inport
  Fault_2 : Inport  Port=2
  Add : Sum
  Add1 : Sum
  Gain : Gain  Gain=Gain_Beta_2_m2
  Random Number : RandomNumber  Mean=m_Beta  Variance=sigma_Beta  Seed=seed(10)  SampleTime=Ts
  Random Number1 : RandomNumber  Mean=m_Beta  Variance=sigma_Beta  Seed=seed(11)  SampleTime=Ts
  Switch : Switch  Threshold=.5
  Beta_2_m1 : Outport
  Beta_2_m2 : Outport  Port=2
  wires:
  Random Number1/1 -> Add1/2
  Random Number/1 -> Add/1
  Beta_2/1 -> Add1/1, Add/2
  Add/1 -> Beta_2_m1/1
  Add1/1 -> Switch/1, Gain/1
  Gain/1 -> Switch/3
  Switch/1 -> Beta_2_m2/1
  Fault_2/1 -> Switch/2

== system FDIBenchMark/Sensors/Pitch3 Sensor ==
  Beta_3 : Inport
  Fault_3 : Inport  Port=2
  Add : Sum
  Add1 : Sum
  Constant : Constant  Value=Constant_Beta_3_m1
  Random Number : RandomNumber  Mean=m_Beta  Variance=sigma_Beta  Seed=seed(12)  SampleTime=Ts
  Random Number1 : RandomNumber  Mean=m_Beta  Variance=sigma_Beta  Seed=seed(13)  SampleTime=Ts
  Switch : Switch  Threshold=0.5
  Beta_3_m1 : Outport
  Beta_3_m2 : Outport  Port=2
  wires:
  Random Number1/1 -> Add1/2
  Add1/1 -> Beta_3_m2/1
  Random Number/1 -> Add/1
  Beta_3/1 -> Add1/1, Add/2
  Fault_3/1 -> Switch/2
  Constant/1 -> Switch/3
  Add/1 -> Switch/1
  Switch/1 -> Beta_3_m1/1

== system FDIBenchMark/Sensors/Tau_g Sensor ==
  Tau_g : Inport
  Add : Sum
  Random Number : RandomNumber  Mean=m_tau_g  Variance=sigma_tau_g  Seed=seed(6)  SampleTime=Ts
  Tau_g_m : Outport
  wires:
  Add/1 -> Tau_g_m/1
  Tau_g/1 -> Add/1
  Random Number/1 -> Add/2

== system FDIBenchMark/Sensors/Wind Sensor ==
  v_hub : Inport
  Add : Sum
  Random Number : RandomNumber  Mean=m_vw  Variance=sigma_vm  Seed=seed(1)  SampleTime=Ts
  v_hub_m : Outport
  wires:
  Random Number/1 -> Add/2
  v_hub/1 -> Add/1
  Add/1 -> v_hub_m/1

== system FDIBenchMark/Wind model/3rd_Harmonic_Filter1 ==
  avg_wind : Inport
  in_1 : Inport  Port=2
  3rd harmonic Filter : Subsystem
  Unit Delay : UnitDelay  SampleTime=T_sample
  out_1 : Outport
  wires:
  3rd harmonic Filter/1(Out) -> out_1/1
  avg_wind/1 -> 3rd harmonic Filter/1(avg_wind)
  in_1/1 -> Unit Delay/1
  Unit Delay/1 -> 3rd harmonic Filter/2(In)

== system FDIBenchMark/Wind model/Kaimal_Filter_1 ==
  in_1 : Inport
  avg_wind : Inport  Port=2
  Fcn : Fcn  Expr=turb_int*sqrt(L*u(1))/100/sqrt(2)
  Kaimal Filter : Subsystem
  Product : Product  SaturateOnIntegerOverflow=on  OutDataTypeStr=Inherit: Same as first input
  Unit Delay : UnitDelay  SampleTime=T_sample
  out_1 : Outport
  wires:
  Product/1 -> out_1/1
  Kaimal Filter/1(Out) -> Product/2
  Fcn/1 -> Product/1
  avg_wind/1 -> Fcn/1, Kaimal Filter/1(avg_wind)
  in_1/1 -> Unit Delay/1
  Unit Delay/1 -> Kaimal Filter/2(In)

== system FDIBenchMark/Wind model/Kaimal_Filter_2 ==
  avg_wind : Inport
  in_1 : Inport  Port=2
  Fcn : Fcn  Expr=turb_int*sqrt(L*u(1))/100/sqrt(2)
  Kaimal Filter : Subsystem
  Product : Product  SaturateOnIntegerOverflow=on  OutDataTypeStr=Inherit: Same as first input
  Unit Delay : UnitDelay  SampleTime=T_sample
  out_1 : Outport
  wires:
  Unit Delay/1 -> Kaimal Filter/2(In)
  in_1/1 -> Unit Delay/1
  avg_wind/1 -> Kaimal Filter/1(avg_wind), Fcn/1
  Fcn/1 -> Product/1
  Kaimal Filter/1(Out) -> Product/2
  Product/1 -> out_1/1

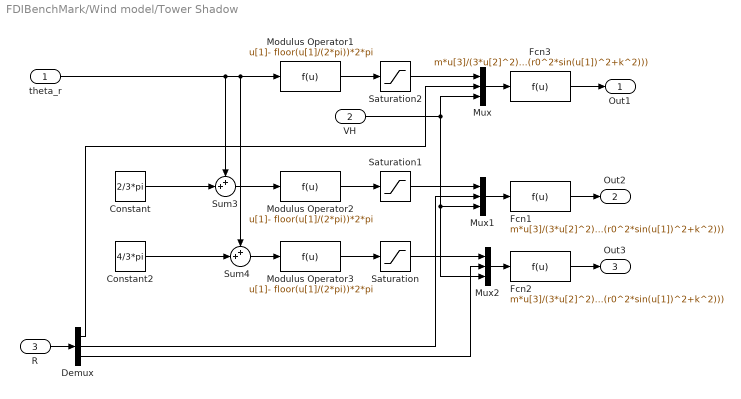
== system FDIBenchMark/Wind model/Tower Shadow ==
  theta_r : Inport
  VH : Inport  Port=2
  R : Inport  Port=3
  Constant : Constant  Value=2/3*pi
  Constant2 : Constant  Value=4/3*pi
  Demux : Demux  Outputs=3
  Fcn1 : Fcn  Expr=m*u[3]/(3*u[2]^2)*(a^2*2*(u[2]^2-r0^2)/((u[2]^2+r0^2)*sin(u[1])^2+2*k^2)+2*a^2*k^2*(r0^2-u[2]^2)/((u[2]^2*sin(u[1])^2+k^2)*(r0^2*sin(u[1])^2+k^2)))
  Fcn2 : Fcn  Expr=m*u[3]/(3*u[2]^2)*(a^2*2*(u[2]^2-r0^2)/((u[2]^2+r0^2)*sin(u[1])^2+2*k^2)+2*a^2*k^2*(r0^2-u[2]^2)/((u[2]^2*sin(u[1])^2+k^2)*(r0^2*sin(u[1])^2+k^2)))
  Fcn3 : Fcn  Expr=m*u[3]/(3*u[2]^2)*(a^2*2*(u[2]^2-r0^2)/((u[2]^2+r0^2)*sin(u[1])^2+2*k^2)+2*a^2*k^2*(r0^2-u[2]^2)/((u[2]^2*sin(u[1])^2+k^2)*(r0^2*sin(u[1])^2+k^2)))
  Modulus Operator1 : Fcn  Expr=u[1]- floor(u[1]/(2*pi))*2*pi
  Modulus Operator2 : Fcn  Expr=u[1]- floor(u[1]/(2*pi))*2*pi
  Modulus Operator3 : Fcn  Expr=u[1]- floor(u[1]/(2*pi))*2*pi
  Mux : Mux  Inputs=3
  Mux1 : Mux  Inputs=3
  Mux2 : Mux  Inputs=3
  Saturation : Saturate  UpperLimit=3*pi/2  LowerLimit=pi/2
  Saturation1 : Saturate  UpperLimit=3*pi/2  LowerLimit=pi/2
  Saturation2 : Saturate  UpperLimit=3*pi/2  LowerLimit=pi/2
  Sum3 : Sum  Inputs=++|
  Sum4 : Sum  Inputs=++|
  Out1 : Outport
  Out2 : Outport  Port=2
  Out3 : Outport  Port=3
  wires:
  theta_r/1 -> Sum3/1, Sum4/1, Modulus Operator1/1
  Sum4/1 -> Modulus Operator3/1
  Constant2/1 -> Sum4/2
  Sum3/1 -> Modulus Operator2/1
  Constant/1 -> Sum3/2
  Modulus Operator1/1 -> Saturation2/1
  Modulus Operator2/1 -> Saturation1/1
  Modulus Operator3/1 -> Saturation/1
  Mux/1 -> Fcn3/1
  Saturation2/1 -> Mux/1
  Demux/1 -> Mux/2
  R/1 -> Demux/1
  Mux1/1 -> Fcn1/1
  Saturation1/1 -> Mux1/1
  Demux/2 -> Mux1/2
  Mux2/1 -> Fcn2/1
  Saturation/1 -> Mux2/1
  Demux/3 -> Mux2/2
  VH/1 -> Mux/3, Mux2/3, Mux1/3
  Fcn3/1 -> Out1/1
  Fcn1/1 -> Out2/1
  Fcn2/1 -> Out3/1

== system FDIBenchMark/Wind model/White Noise_1 ==
  Gain : Gain  Gain=[sqrt(Cov)]/[sqrt(Ts)]  SaturateOnIntegerOverflow=on  OutDataTypeStr=Inherit: Same as input  ParamDataTypeStr=Inherit: Same as input
  White Noise : RandomNumber  Seed=seed  SampleTime=Ts
  Zero-Order Hold : ZeroOrderHold  SampleTime=Ts
  Out_1 : Outport
  wires:
  White Noise/1 -> Zero-Order Hold/1
  Gain/1 -> Out_1/1
  Zero-Order Hold/1 -> Gain/1

== system FDIBenchMark/Wind model/White Noise_2 ==
  Gain : Gain  Gain=[sqrt(Cov)]/[sqrt(Ts)]  SaturateOnIntegerOverflow=on  OutDataTypeStr=Inherit: Same as input  ParamDataTypeStr=Inherit: Same as input
  White Noise : RandomNumber  Seed=seed  SampleTime=Ts
  Zero-Order Hold : ZeroOrderHold  SampleTime=Ts
  Out_1 : Outport
  wires:
  White Noise/1 -> Zero-Order Hold/1
  Gain/1 -> Out_1/1
  Zero-Order Hold/1 -> Gain/1

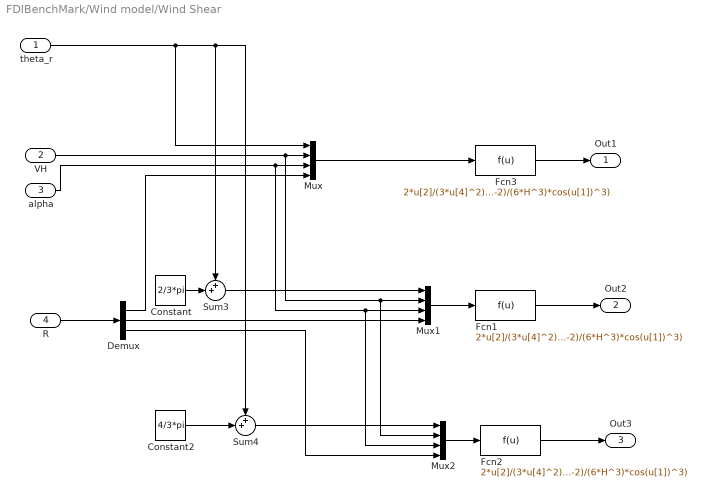
== system FDIBenchMark/Wind model/Wind Shear ==
  theta_r : Inport
  VH : Inport  Port=2
  alpha : Inport  Port=3
  R : Inport  Port=4
  Constant : Constant  Value=2/3*pi
  Constant2 : Constant  Value=4/3*pi
  Demux : Demux  Outputs=3
  Fcn1 : Fcn  Expr=2*u[2]/(3*u[4]^2)*(u[4]^3/3*u[3]/H*cos(u[1])+u[4]^4/4*u[3]*(u[3]-1)/(2*H^2)*cos(u[1])^2+u[4]^5/5*u[3]*(u[3]-1)*(u[3]-2)/(6*H^3)*cos(u[1])^3)
  Fcn2 : Fcn  Expr=2*u[2]/(3*u[4]^2)*(u[4]^3/3*u[3]/H*cos(u[1])+u[4]^4/4*u[3]*(u[3]-1)/(2*H^2)*cos(u[1])^2+u[4]^5/5*u[3]*(u[3]-1)*(u[3]-2)/(6*H^3)*cos(u[1])^3)
  Fcn3 : Fcn  Expr=2*u[2]/(3*u[4]^2)*(u[4]^3/3*u[3]/H*cos(u[1])+u[4]^4/4*u[3]*(u[3]-1)/(2*H^2)*cos(u[1])^2+u[4]^5/5*u[3]*(u[3]-1)*(u[3]-2)/(6*H^3)*cos(u[1])^3)
  Mux : Mux
  Mux1 : Mux
  Mux2 : Mux
  Sum3 : Sum  Inputs=++|
  Sum4 : Sum  Inputs=++|
  Out1 : Outport
  Out2 : Outport  Port=2
  Out3 : Outport  Port=3
  wires:
  theta_r/1 -> Sum3/1, Sum4/1, Mux/1
  VH/1 -> Mux/2, Mux1/2, Mux2/2
  Sum4/1 -> Mux2/1
  Constant2/1 -> Sum4/2
  Sum3/1 -> Mux1/1
  Constant/1 -> Sum3/2
  alpha/1 -> Mux/3, Mux1/3, Mux2/3
  Fcn2/1 -> Out3/1
  Fcn1/1 -> Out2/1
  Mux/1 -> Fcn3/1
  R/1 -> Demux/1
  Demux/1 -> Mux/4
  Mux1/1 -> Fcn1/1
  Mux2/1 -> Fcn2/1
  Demux/2 -> Mux1/4
  Demux/3 -> Mux2/4
  Fcn3/1 -> Out1/1

== system FDIBenchMark/Wind model/ZERO_Harmonic_Filter ==
  in_1 : Inport
  avg_wind : Inport  Port=2
  Unit Delay : UnitDelay  SampleTime=T_sample
  ZERO harmonic Filter : Subsystem
  out_1 : Outport
  wires:
  Unit Delay/1 -> ZERO harmonic Filter/2(In)
  in_1/1 -> Unit Delay/1
  avg_wind/1 -> ZERO harmonic Filter/1(avg_wind)
  ZERO harmonic Filter/1(Out) -> out_1/1

== system FDIBenchMark/Blade&Pitch System/Pitch Systems/PitchSystem 1 ==
  Beta_r : Inport
  Transfer Fcn : TransferFcn  Numerator=[omega_n^2]  Denominator=[1 2*xi*omega_n omega_n^2]
  Beta_1 : Outport
  wires:
  Beta_r/1 -> Transfer Fcn/1
  Transfer Fcn/1 -> Beta_1/1

== system FDIBenchMark/Blade&Pitch System/Pitch Systems/PitchSystem 2 ==
  Beta_r : Inport
  Fault_6 : Inport  Port=2
  Add : Sum
  Gain : Gain  Gain=Apb  Multiplication=Matrix(K*u)
  Gain1 : Gain  Gain=Bpb  Multiplication=Matrix(K*u)
  Gain2 : Gain  Gain=Cpb  Multiplication=Matrix(K*u)
  Gain3 : Gain  Gain=Apb1  Multiplication=Matrix(K*u)
  Gain4 : Gain  Gain=Bpb1  Multiplication=Matrix(K*u)
  Gain5 : Gain  Gain=Cpb1  Multiplication=Matrix(K*u)
  Integrator : Integrator
  Switch1 : Switch  Threshold=0.5
  Switch2 : Switch  Threshold=0.5
  Switch3 : Switch  Threshold=0.5
  Beta_2 : Outport
  wires:
  Integrator/1 -> Gain/1, Gain3/1, Gain2/1, Gain5/1
  Add/1 -> Integrator/1
  Switch1/1 -> Add/1
  Gain1/1 -> Switch1/1
  Gain4/1 -> Switch1/3
  Gain/1 -> Switch2/1
  Gain3/1 -> Switch2/3
  Switch2/1 -> Add/2
  Fault_6/1 -> Switch1/2, Switch2/2, Switch3/2
  Beta_r/1 -> Gain1/1, Gain4/1
  Gain2/1 -> Switch3/1
  Switch3/1 -> Beta_2/1
  Gain5/1 -> Switch3/3

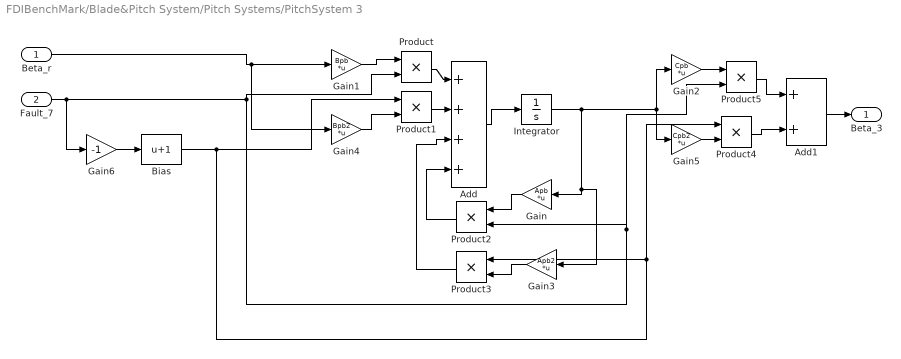
== system FDIBenchMark/Blade&Pitch System/Pitch Systems/PitchSystem 3 ==
  Beta_r : Inport
  Fault_7 : Inport  Port=2
  Add : Sum  Inputs=++++
  Add1 : Sum
  Bias : Bias  Bias=1
  Gain : Gain  Gain=Apb  Multiplication=Matrix(K*u)
  Gain1 : Gain  Gain=Bpb  Multiplication=Matrix(K*u)
  Gain2 : Gain  Gain=Cpb  Multiplication=Matrix(K*u)
  Gain3 : Gain  Gain=Apb2  Multiplication=Matrix(K*u)
  Gain4 : Gain  Gain=Bpb2  Multiplication=Matrix(K*u)
  Gain5 : Gain  Gain=Cpb2  Multiplication=Matrix(K*u)
  Gain6 : Gain  Gain=-1
  Integrator : Integrator
  Product{,1..5} (6 alike) : Product  RndMeth=Zero
  Beta_3 : Outport
  wires:
  Beta_r/1 -> Gain4/1, Gain1/1
  Fault_7/1 -> Product2/2, Product5/2, Product/2, Gain6/1
  Gain4/1 -> Product1/2
  Add/1 -> Integrator/1
  Integrator/1 -> Gain5/1, Gain2/1, Gain3/1, Gain/1
  Product/1 -> Add/1
  Gain1/1 -> Product/1
  Product1/1 -> Add/2
  Gain3/1 -> Product3/2
  Gain/1 -> Product2/1
  Product2/1 -> Add/4
  Product3/1 -> Add/3
  Add1/1 -> Beta_3/1
  Gain2/1 -> Product5/1
  Gain5/1 -> Product4/2
  Product4/1 -> Add1/2
  Product5/1 -> Add1/1
  Gain6/1 -> Bias/1
  Bias/1 -> Product1/1, Product3/1, Product4/1

== system FDIBenchMark/Blade&Pitch System/Subsystem/AeroDyn 1 ==
  v_w : Inport
  Omega_r : Inport  Port=2
  Beta_1 : Inport  Port=3
  Divide : Product  Inputs=/*
  Divide1 : Product  Inputs=***
  Gain : Gain  Gain=R
  Gain1 : Gain  Gain=rho*pi*R^3/6
  Lookup Table (2-D) : Lookup2D  RowIndex=Lambda  ColumnIndex=Angle  Table=Cq
  Tau_r1 : Outport
  wires:
  Divide/1 -> Lookup Table (2-D)/1
  Gain/1 -> Divide/2
  v_w/1 -> Divide/1, Divide1/2, Divide1/1
  Lookup Table (2-D)/1 -> Divide1/3
  Divide1/1 -> Gain1/1
  Omega_r/1 -> Gain/1
  Gain1/1 -> Tau_r1/1
  Beta_1/1 -> Lookup Table (2-D)/2

== system FDIBenchMark/Blade&Pitch System/Subsystem/AeroDyn 2 ==
  v_w : Inport
  Omega_r : Inport  Port=2
  Beta_2 : Inport  Port=3
  Divide : Product  Inputs=/*
  Divide1 : Product  Inputs=***
  Gain : Gain  Gain=R
  Gain1 : Gain  Gain=rho*pi*R^3/6
  Lookup Table (2-D) : Lookup2D  RowIndex=Lambda  ColumnIndex=Angle  Table=Cq
  Tau_r2 : Outport
  wires:
  Beta_2/1 -> Lookup Table (2-D)/2
  Gain1/1 -> Tau_r2/1
  Omega_r/1 -> Gain/1
  Divide1/1 -> Gain1/1
  Lookup Table (2-D)/1 -> Divide1/3
  v_w/1 -> Divide1/1, Divide1/2, Divide/1
  Gain/1 -> Divide/2
  Divide/1 -> Lookup Table (2-D)/1

== system FDIBenchMark/Blade&Pitch System/Subsystem/AeroDyn 3 ==
  v_w : Inport
  Omega_r : Inport  Port=2
  Beta_3 : Inport  Port=3
  Divide : Product  Inputs=/*
  Divide1 : Product  Inputs=***
  Gain : Gain  Gain=R
  Gain1 : Gain  Gain=rho*pi*R^3/6
  Lookup Table (2-D) : Lookup2D  RowIndex=Lambda  ColumnIndex=Angle  Table=Cq
  Tau_r3 : Outport
  wires:
  Divide/1 -> Lookup Table (2-D)/1
  Gain/1 -> Divide/2
  v_w/1 -> Divide/1, Divide1/2, Divide1/1
  Lookup Table (2-D)/1 -> Divide1/3
  Divide1/1 -> Gain1/1
  Omega_r/1 -> Gain/1
  Gain1/1 -> Tau_r3/1
  Beta_3/1 -> Lookup Table (2-D)/2

== system FDIBenchMark/Detectie Anomalii/Detectie Fault_1/Calcul FFT ==
  Intrare_Semnal : Inport
  MATLAB Function : MATLAB Function  TreatAsAtomicUnit=on  SystemSampleTime=Ts * (Lungime_Fereastra / 4)
  MATLAB Function1 : MATLAB Function  TreatAsAtomicUnit=on  SystemSampleTime=Ts * (Lungime_Fereastra / 4)
  Matrix Concatenate : Concatenate  Mode=Multidimensional array  ConcatenateDimension=2
  Iesire_Matrice : Outport
  wires:
  MATLAB Function1/1(y) -> MATLAB Function/1(u)
  MATLAB Function/1(y_magnitudine) -> Matrix Concatenate/1
  MATLAB Function/2(y_frecventa) -> Matrix Concatenate/2
  Intrare_Semnal/1 -> MATLAB Function1/1(u)
  Matrix Concatenate/1 -> Iesire_Matrice/1

== system FDIBenchMark/Detectie Anomalii/Detectie Fault_1/Calcul Medie ==
  Intrare_Semnal : Inport
  MATLAB Function : MATLAB Function  TreatAsAtomicUnit=on  SystemSampleTime=Ts * Lungime_Fereastra_2
  Iesire_Valoare : Outport
  wires:
  Intrare_Semnal/1 -> MATLAB Function/1(u)
  MATLAB Function/1(y) -> Iesire_Valoare/1

== system FDIBenchMark/Detectie Anomalii/Detectie Fault_1/Decizie Fault_1 ==
  Intrare_Valoare_Medie : Inport
  Intrare_Matrice_FFT : Inport  Port=2
  Delay : Delay  DelayLength=1  InitialCondition=0  SampleTime=Ts * Lungime_Fereastra_2
  Delay1 : Delay  InitialCondition=0  SampleTime=Ts * Lungime_Fereastra_2
  MATLAB Function : MATLAB Function  TreatAsAtomicUnit=on  SystemSampleTime=Ts
  MATLAB Function1 : MATLAB Function  TreatAsAtomicUnit=on  SystemSampleTime=Ts * Lungime_Fereastra_2
  MATLAB Function2 : MATLAB Function  TreatAsAtomicUnit=on  SystemSampleTime=Ts * (Lungime_Fereastra / 4)
  Scope_Decizie_FFT : Scope
      settings: YMin=-0  YMax=2  SaveName=ScopeData3
  Scope_Decizie_Fault_1 : Scope
      settings: SaveName=ScopeData7
  Scope_Decizie_Medie : Scope
      settings: YMin=0  YMax=1  SaveName=ScopeData2
  To Workspace : ToWorkspace  VariableName=Decizie_Medie_Fault_1  SaveFormat=Structure With Time  SampleTime=Ts
  To Workspace1 : ToWorkspace  VariableName=Decizie_FFT_Fault_1  SaveFormat=Structure With Time  SampleTime=Ts
  To Workspace2 : ToWorkspace  VariableName=Decizie_Fault_1  SaveFormat=Structure With Time  SampleTime=Ts
  Iesire_Decizie : Outport
  wires:
  Intrare_Matrice_FFT/1 -> MATLAB Function2/1(u)
  MATLAB Function/1(y) -> Iesire_Decizie/1, To Workspace2/1, Scope_Decizie_Fault_1/1
  MATLAB Function2/1(y) -> To Workspace1/1, Scope_Decizie_FFT/1, MATLAB Function/2(u2)
  Intrare_Valoare_Medie/1 -> Delay1/1, Delay/1, MATLAB Function1/1(u)
  Delay/1 -> MATLAB Function1/2(u1)
  Delay1/1 -> MATLAB Function1/3(u2)
  MATLAB Function1/1(y) -> Scope_Decizie_Medie/1, To Workspace/1, MATLAB Function/1(u1)

== system FDIBenchMark/Detectie Anomalii/Detectie Fault_1/Ferestruire Semnal ==
  note: Tipul ferestrei: Dreptunghiulară
      | Lungimea ferestre: Lungime_fereastra_2
      | Factor de suprapunere: 0%
  Intrare_Semnal : Inport
  Buffer : Buffer  N=Lungime_Fereastra_2  TreatMby1Signals=One channel
  Zero-Order Hold : ZeroOrderHold  SampleTime=Ts
  Iesire_Semnal : Outport
  wires:
  Buffer/1 -> Iesire_Semnal/1
  Intrare_Semnal/1 -> Zero-Order Hold/1
  Zero-Order Hold/1 -> Buffer/1

== system FDIBenchMark/Detectie Anomalii/Detectie Fault_1/Ferestruire si Suprapunere Semnal ==
  note: Tipul ferestrei: Dreptunghiulară
      | Lungimea ferestre: Lungime_fereastra
      | Factor de suprapunere: 75%
  Intrare_Semnal : Inport
  Buffer : Buffer  N=Lungime_Fereastra / 4  TreatMby1Signals=One channel
  Delay1 : Delay  DelayLength=Lungime_Fereastra / 4  InitialCondition=0  InputProcessing=Columns as channels (frame based)  SampleTime=Ts
  Delay2 : Delay  DelayLength=Lungime_Fereastra / 4 * 2  InitialCondition=0  InputProcessing=Columns as channels (frame based)  SampleTime=Ts
  Delay3 : Delay  DelayLength=Lungime_Fereastra / 4 * 3  InitialCondition=0  InputProcessing=Columns as channels (frame based)  SampleTime=Ts
  Matrix Concatenate : Concatenate  NumInputs=4  Mode=Multidimensional array
  Zero-Order Hold : ZeroOrderHold  SampleTime=Ts
  Iesire_Semnal : Outport
  wires:
  Delay3/1 -> Matrix Concatenate/1
  Matrix Concatenate/1 -> Iesire_Semnal/1
  Buffer/1 -> Delay2/1, Delay3/1, Matrix Concatenate/4, Delay1/1
  Intrare_Semnal/1 -> Zero-Order Hold/1
  Zero-Order Hold/1 -> Buffer/1
  Delay1/1 -> Matrix Concatenate/3
  Delay2/1 -> Matrix Concatenate/2

== system FDIBenchMark/Detectie Anomalii/Detectie Fault_3/Calcul FFT ==
  Intrare_Semnal : Inport
  MATLAB Function : MATLAB Function  TreatAsAtomicUnit=on  SystemSampleTime=Ts * (Lungime_Fereastra / 4)
  MATLAB Function1 : MATLAB Function  TreatAsAtomicUnit=on  SystemSampleTime=Ts * (Lungime_Fereastra / 4)
  Matrix Concatenate : Concatenate  Mode=Multidimensional array  ConcatenateDimension=2
  Iesire_Matrice : Outport
  wires:
  MATLAB Function1/1(y) -> MATLAB Function/1(u)
  MATLAB Function/1(y_magnitudine) -> Matrix Concatenate/1
  MATLAB Function/2(y_frecventa) -> Matrix Concatenate/2
  Intrare_Semnal/1 -> MATLAB Function1/1(u)
  Matrix Concatenate/1 -> Iesire_Matrice/1

== system FDIBenchMark/Detectie Anomalii/Detectie Fault_3/Calcul Medie ==
  Intrare_Semnal : Inport
  MATLAB Function : MATLAB Function  TreatAsAtomicUnit=on  SystemSampleTime=Ts * Lungime_Fereastra_2
  Iesire_Valoare : Outport
  wires:
  Intrare_Semnal/1 -> MATLAB Function/1(u)
  MATLAB Function/1(y) -> Iesire_Valoare/1

== system FDIBenchMark/Detectie Anomalii/Detectie Fault_3/Decizie Fault_3 ==
  Intrare_Valoare_Medie : Inport
  Intrare_Matrice_FFT : Inport  Port=2
  Delay : Delay  DelayLength=1  InitialCondition=0  SampleTime=Ts * Lungime_Fereastra_2
  Delay1 : Delay  InitialCondition=0  SampleTime=Ts * Lungime_Fereastra_2
  MATLAB Function : MATLAB Function  TreatAsAtomicUnit=on  SystemSampleTime=Ts
  MATLAB Function1 : MATLAB Function  TreatAsAtomicUnit=on  SystemSampleTime=Ts * Lungime_Fereastra_2
  MATLAB Function2 : MATLAB Function  TreatAsAtomicUnit=on  SystemSampleTime=Ts * (Lungime_Fereastra / 4)
  Scope_Decizie_FFT : Scope
      settings: YMin=-0  YMax=2  SaveName=ScopeData3
  Scope_Decizie_Fault_3 : Scope
      settings: SaveName=ScopeData7
  Scope_Decizie_Medie : Scope
      settings: YMin=0  YMax=1  SaveName=ScopeData2
  To Workspace : ToWorkspace  VariableName=Decizie_Medie_Fault_3  SaveFormat=Structure With Time  SampleTime=Ts
  To Workspace1 : ToWorkspace  VariableName=Decizie_FFT_Fault_3  SaveFormat=Structure With Time  SampleTime=Ts
  To Workspace2 : ToWorkspace  VariableName=Decizie_Fault_3  SaveFormat=Structure With Time  SampleTime=Ts
  Iesire_Decizie : Outport
  wires:
  Intrare_Matrice_FFT/1 -> MATLAB Function2/1(u)
  MATLAB Function/1(y) -> Iesire_Decizie/1, To Workspace2/1, Scope_Decizie_Fault_3/1
  MATLAB Function2/1(y) -> To Workspace1/1, Scope_Decizie_FFT/1, MATLAB Function/2(u2)
  Intrare_Valoare_Medie/1 -> Delay1/1, Delay/1, MATLAB Function1/1(u)
  Delay/1 -> MATLAB Function1/2(u1)
  Delay1/1 -> MATLAB Function1/3(u2)
  MATLAB Function1/1(y) -> Scope_Decizie_Medie/1, To Workspace/1, MATLAB Function/1(u1)

== system FDIBenchMark/Detectie Anomalii/Detectie Fault_3/Ferestruire Semnal ==
  note: Tipul ferestrei: Dreptunghiulară
      | Lungimea ferestre: Lungime_fereastra_2
      | Factor de suprapunere: 0%
  Intrare_Semnal : Inport
  Buffer : Buffer  N=Lungime_Fereastra_2  TreatMby1Signals=One channel
  Zero-Order Hold : ZeroOrderHold  SampleTime=Ts
  Iesire_Semnal : Outport
  wires:
  Buffer/1 -> Iesire_Semnal/1
  Intrare_Semnal/1 -> Zero-Order Hold/1
  Zero-Order Hold/1 -> Buffer/1
